simulink model "cartesiano_sim"  (R2013a)
settings: Solver=ode3  StartTime=0.0  StopTime=6  FixedStep=Tm  MaxStep=1e-2  RelTol=1e-3
values from neighbouring files (symbols this model uses):
  Kp = (2*pi*5)^2*eye(3)    [cartesiano_var.m]    (also in hibrido_var.m)
  Kv = 2*sqrt(Kp)*eye(3)    [cartesiano_var.m]    (also in hibrido_var.m)
  q0 = [pi;1/4*pi]    [cartesiano_var.m]    (also in fuerzas_var.m = [0;pi/2]; hibrido_var.m = [0;pi/2])
  robotTP = robotRR    [cartesiano_var.m]    (also in fuerzas_var.m; hibrido_var.m)
undefined symbols (not defined in the file or in its folder): jacob0, modelAlpha, modelBeta
undefined symbols (not defined in the file): robotPlanta
libraries: roblocks x2
settings Model: Creator=Nicola  LastModifiedBy=Nicola

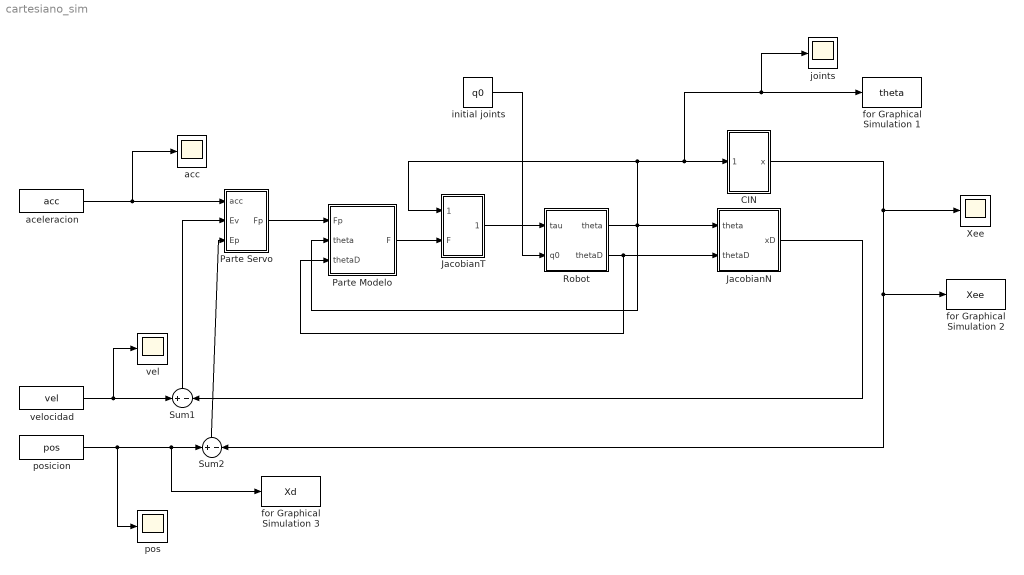
== system cartesiano_sim ==
  CIN : Subsystem
  JacobianN : Subsystem
  JacobianT : Subsystem
  Parte Modelo : Subsystem
  Parte Servo : Subsystem
  Robot : Subsystem
  Sum1 : Sum  Inputs=+|-
  Sum2 : Sum  Inputs=+|-
  Xee : Scope
      settings: TimeRange=7  YMin=-1.5  YMax=1.25
  acc : Scope
      settings: TimeRange=7  YMin=-9.5e-08  YMax=0  SaveName=ScopeData4
  aceleracion : FromWorkspace  VariableName=acc  SampleTime=0
  for Graphical Simulation 1 : ToWorkspace  VariableName=theta  SampleTime=-1  SaveFormat=Timeseries
  for Graphical Simulation 2 : ToWorkspace  VariableName=Xee  SampleTime=-1  SaveFormat=Timeseries
  for Graphical Simulation 3 : ToWorkspace  VariableName=Xd  SampleTime=-1  SaveFormat=Timeseries
  initial joints : Constant  Value=q0
  joints : Scope
      settings: TimeRange=15  YMin=-2  YMax=3.25
  pos : Scope
      settings: TimeRange=7  YMin=0  YMax=7e-09  SaveName=ScopeData3
  posicion : FromWorkspace  VariableName=pos  SampleTime=0
  vel : Scope
      settings: TimeRange=7  YMin=0  YMax=7e-09  SaveName=ScopeData2
  velocidad : FromWorkspace  VariableName=vel  SampleTime=0
  wires:
  Robot/2(thetaD) -> Parte Modelo/3(thetaD), JacobianN/2(thetaD)
  JacobianN/1(xD) -> Sum1/2
  posicion/1 -> pos/1, for Graphical Simulation 3/1, Sum2/1
  velocidad/1 -> vel/1, Sum1/1
  aceleracion/1 -> Parte Servo/1(acc), acc/1
  initial joints/1 -> Robot/2(q0)
  Sum1/1 -> Parte Servo/2(Ev)
  Sum2/1 -> Parte Servo/3(Ep)
  JacobianT/1(tau) -> Robot/1(tau)
  Robot/1(theta) -> Parte Modelo/2(theta), JacobianN/1(theta), JacobianT/1(theta), CIN/1(theta), joints/1, for Graphical Simulation 1/1
  Parte Servo/1(Fp) -> Parte Modelo/1(Fp)
  CIN/1(x) -> for Graphical Simulation 2/1, Sum2/2, Xee/1
  Parte Modelo/1(F) -> JacobianT/2(F)

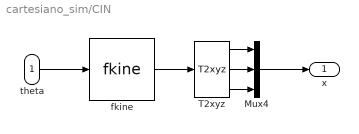
== system cartesiano_sim/CIN ==
  theta : Inport
  Mux4 : Mux  Inputs=3
  T2xyz : roblocks/Transform Conversion/T2xyz
  fkine : roblocks/Kinematics/fkine  robot=robotTP.links
  x : Outport
  wires:
  T2xyz/1 -> Mux4/1
  T2xyz/3 -> Mux4/3
  Mux4/1 -> x/1
  T2xyz/2 -> Mux4/2
  theta/1 -> fkine/1
  fkine/1 -> T2xyz/1

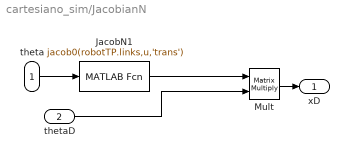
== system cartesiano_sim/JacobianN ==
  theta : Inport
  thetaD : Inport  Port=2
  JacobN1 : MATLABFcn  MATLABFcn=jacob0(robotTP.links,u,'trans')  OutputDimensions=[3,2]  Output1D=off
  Mult : Product  Multiplication=Matrix(*)
  xD : Outport
  wires:
  Mult/1 -> xD/1
  thetaD/1 -> Mult/2
  JacobN1/1 -> Mult/1
  theta/1 -> JacobN1/1

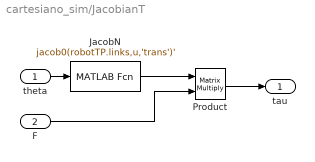
== system cartesiano_sim/JacobianT ==
  theta : Inport
  F : Inport  Port=2
  JacobN : MATLABFcn  MATLABFcn=jacob0(robotTP.links,u,'trans')'  OutputDimensions=[2,3]  Output1D=off
  Product : Product  Multiplication=Matrix(*)
  tau : Outport
  wires:
  theta/1 -> JacobN/1
  JacobN/1 -> Product/1
  F/1 -> Product/2
  Product/1 -> tau/1

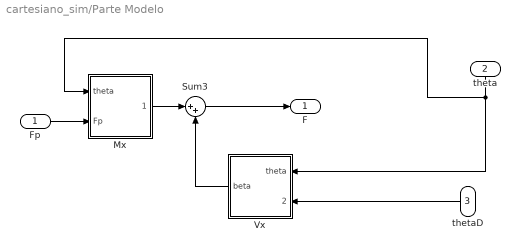
== system cartesiano_sim/Parte Modelo ==
  Fp : Inport
  theta : Inport  Port=2
  thetaD : Inport  Port=3
  Mx : Subsystem
  Sum3 : Sum  Inputs=|++
  Vx : Subsystem
  F : Outport
  wires:
  Fp/1 -> Mx/2(Fp)
  thetaD/1 -> Vx/2(thetaD)
  theta/1 -> Mx/1(theta), Vx/1(theta)
  Mx/1(alpha*F) -> Sum3/1
  Vx/1(beta) -> Sum3/2
  Sum3/1 -> F/1

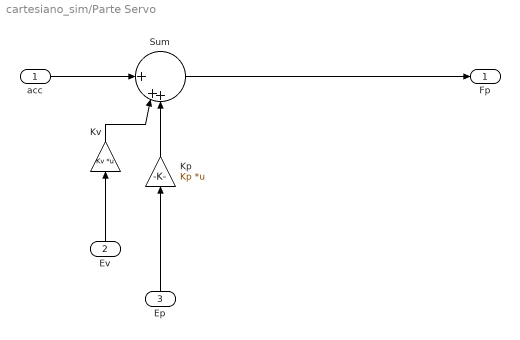
== system cartesiano_sim/Parte Servo ==
  acc : Inport
  Ev : Inport  Port=2
  Ep : Inport  Port=3
  Kp : Gain  Gain=Kp  Multiplication=Matrix(K*u)
  Kv : Gain  Gain=Kv  Multiplication=Matrix(K*u)
  Sum : Sum  Inputs=||||+||++
  Fp : Outport
  wires:
  acc/1 -> Sum/1
  Ev/1 -> Kv/1
  Kp/1 -> Sum/3
  Ep/1 -> Kp/1
  Kv/1 -> Sum/2
  Sum/1 -> Fp/1

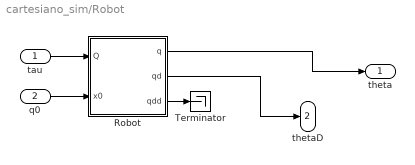
== system cartesiano_sim/Robot ==
  tau : Inport
  q0 : Inport  Port=2
  Robot : Subsystem  AncestorBlock=roblocks/Dynamics/Robot  mask{robot=robotPlanta, q0=[0,0,0,0,0,0]}
      mask prompts: robot "Robot object"; q0 "Initial state"
      mask help: Rigid-body dynamic model of robot.
      mask init:
      | if isa(robot, 'SerialLink')
      |     rname = robot.name;
      |     %fprintf('**robot name is %s\n', rname);
      | else
      |     rname = '';
      |     n = 0
      | end
      mask Help:
      | Simulates the forward (direct) rigid-body dynamics of the robot described
      | by the given robot object.  For given applied joint torque/force it computes
      | the instaneous joint coordinates, velocities and acclerations.
      | 
      | 
      | <b>Parameters::</b>
      | 
      | robot (SerialLink) a dynamic model of an N-link serial link manipulator
      | q0 (1xN)  Initial joint coordinates
      | 
      | <b>Inputs::</b>
      | 
      | Q (1xN) the generalized joint force (torque or force) required to achieve
      | the motion state (q, qd, qdd).
      | 
      | <b>Outputs::</b>
      | 
      | q (1xN) joint coordinates
      | qd (1xN) joint coordinate velocity
      | qdd (1xN) joint coordinate acceleration
      | 
      | 
      | <b>Notes::</b>
      | 
      | - Required to simulate robot rigid body motion.
      | - Implemented using the recursive Newton-Euler scheme (RNE).
      | - A wrapper for the Toolbox method accel() which in turn depends on the
      |   method rne().
      mask Display:
      | port_label('input', 1, 'Q')
      | port_label('output', 1, 'q')
      | port_label('output', 2, 'qd')
      | port_label('output', 3, 'qdd')
      | text(0.1, 0.9,  rname, 'horizontalAlignment', 'left')
  Terminator : Terminator
  theta : Outport
  thetaD : Outport  Port=2
  wires:
  Robot/1(q) -> theta/1
  tau/1 -> Robot/1(Q)
  Robot/3(qdd) -> Terminator/1
  Robot/2(qd) -> thetaD/1
  q0/1 -> Robot/2(x0)

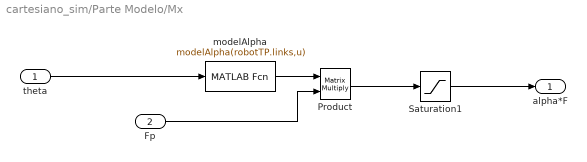
== system cartesiano_sim/Parte Modelo/Mx ==
  theta : Inport
  Fp : Inport  Port=2
  Product : Product  Multiplication=Matrix(*)
  Saturation1 : Saturate  UpperLimit=1e10  LowerLimit=-1e10
  modelAlpha : MATLABFcn  MATLABFcn=modelAlpha(robotTP.links,u)  OutputDimensions=[3,3]  Output1D=off
  alpha*F : Outport
  wires:
  modelAlpha/1 -> Product/1
  Fp/1 -> Product/2
  theta/1 -> modelAlpha/1
  Product/1 -> Saturation1/1
  Saturation1/1 -> alpha*F/1

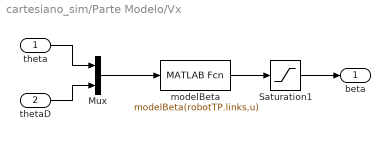
== system cartesiano_sim/Parte Modelo/Vx ==
  theta : Inport
  thetaD : Inport  Port=2
  Mux : Mux  Inputs=2
  Saturation1 : Saturate  UpperLimit=1e3  LowerLimit=-1e3
  modelBeta : MATLABFcn  MATLABFcn=modelBeta(robotTP.links,u)  OutputDimensions=[3,1]  Output1D=off
  beta : Outport
  wires:
  theta/1 -> Mux/1
  thetaD/1 -> Mux/2
  Mux/1 -> modelBeta/1
  modelBeta/1 -> Saturation1/1
  Saturation1/1 -> beta/1

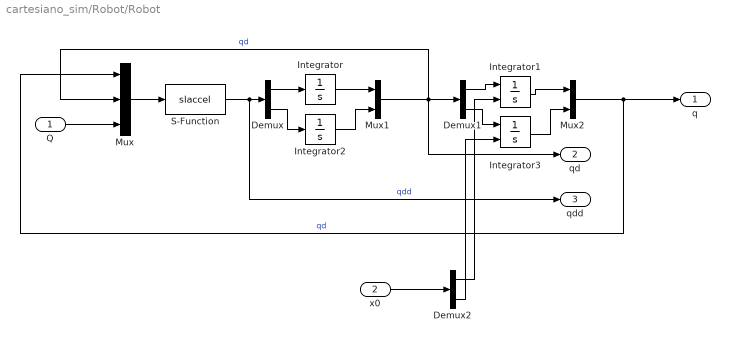
== system cartesiano_sim/Robot/Robot ==
  Q : Inport
  x0 : Inport  Port=2
  Demux : Demux  Outputs=2
  Demux1 : Demux  Outputs=2
  Demux2 : Demux  Outputs=2
  Integrator : Integrator
  Integrator1 : Integrator  InitialConditionSource=external
  Integrator2 : Integrator
  Integrator3 : Integrator  InitialConditionSource=external  InitialCondition=3/4*pi
  Mux : Mux  Inputs=3
  Mux1 : Mux  Inputs=2
  Mux2 : Mux  Inputs=2
  S-Function : S-Function  FunctionName=slaccel  Parameters=robot  EnableBusSupport=off
  q : Outport
  qd : Outport  Port=2
  qdd : Outport  Port=3
  wires:
  Q/1 -> Mux/3
  Mux/1 -> S-Function/1
  S-Function/1 -> Demux/1, qdd/1  "qdd"
  Demux/2 -> Integrator2/1
  Demux/1 -> Integrator/1
  Integrator/1 -> Mux1/1
  Integrator2/1 -> Mux1/2
  Mux1/1 -> Demux1/1, qd/1, Mux/2  "qd"
  Demux1/2 -> Integrator3/1
  Demux1/1 -> Integrator1/1
  Integrator1/1 -> Mux2/1
  Integrator3/1 -> Mux2/2
  Mux2/1 -> Mux/1, q/1  "qd"
  x0/1 -> Demux2/1
  Demux2/1 -> Integrator1/2
  Demux2/2 -> Integrator3/2
